simulink model "NonlinearSystemIdentificationMethod1"  (R2022b)
settings: Solver=VariableStepAuto  StartTime=0.0  StopTime=4  RelTol=0.00001
undefined symbols (not defined in the file): K, L, T, T1, T2
settings Model: Creator=amirz  LastModifiedBy=amirz

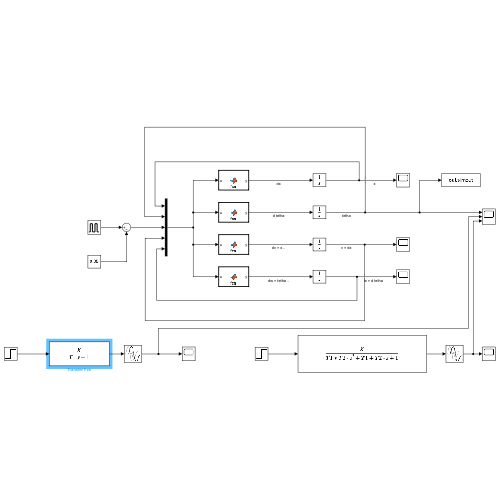
[thumbnail: Simulink's stored preview of the top-level diagram]
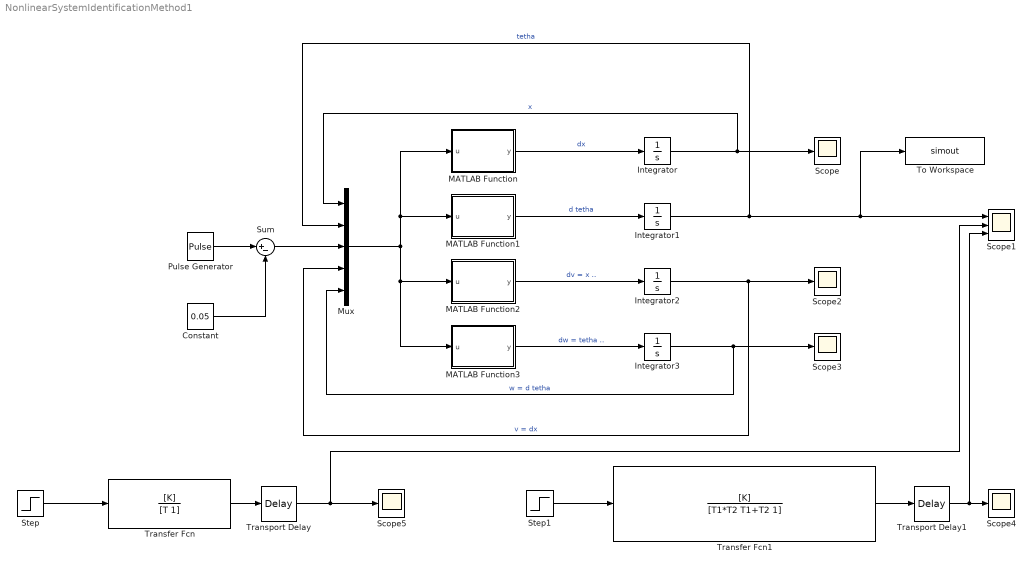
== system NonlinearSystemIdentificationMethod1 ==
  Constant : Constant  Value=0.05
  Integrator{,1..3} (4 alike) : Integrator
  MATLAB Function : MATLAB Function  TreatAsAtomicUnit=on
  MATLAB Function1 : MATLAB Function  TreatAsAtomicUnit=on
  MATLAB Function2 : MATLAB Function  TreatAsAtomicUnit=on
  MATLAB Function3 : MATLAB Function  TreatAsAtomicUnit=on
  Mux : Mux  Inputs=5
  Pulse Generator : DiscretePulseGenerator  PulseType=Time based  Amplitude=-0.1  Period=0.01  PulseWidth=50
  Scope{,2..5} (5 alike) : Scope
  Scope1 : Scope  NumInputPorts=3
  Step : Step  Time=0  SampleTime=0
  Step1 : Step  Time=0  SampleTime=0
  Sum : Sum  Inputs=|+-
  To Workspace : ToWorkspace  VariableName=simout  SaveFormat=Timeseries  SampleTime=-1
  Transfer Fcn : TransferFcn  Numerator=[K]  Denominator=[T 1]
  Transfer Fcn1 : TransferFcn  Numerator=[K]  Denominator=[T1*T2 T1+T2 1]
  Transport Delay : TransportDelay  DelayTime=L  InitialOutput=0.01
  Transport Delay1 : TransportDelay  DelayTime=L
  wires:
  MATLAB Function3/1(y) -> Integrator3/1  "dw = tetha .."
  MATLAB Function2/1(y) -> Integrator2/1  "dv = x .."
  MATLAB Function1/1(y) -> Integrator1/1  "d tetha"
  MATLAB Function/1(y) -> Integrator/1  "dx"
  Integrator3/1 -> Mux/5, Scope3/1  "w = d tetha"
  Integrator2/1 -> Mux/4, Scope2/1  "v = dx"
  Integrator1/1 -> To Workspace/1, Scope1/1, Mux/2  "tetha"
  Integrator/1 -> Mux/1, Scope/1  "x"
  Mux/1 -> MATLAB Function2/1(u), MATLAB Function3/1(u), MATLAB Function/1(u), MATLAB Function1/1(u)
  Transfer Fcn/1 -> Transport Delay/1
  Transfer Fcn1/1 -> Transport Delay1/1
  Step1/1 -> Transfer Fcn1/1
  Transport Delay/1 -> Scope1/2, Scope5/1
  Step/1 -> Transfer Fcn/1
  Sum/1 -> Mux/3
  Pulse Generator/1 -> Sum/1
  Constant/1 -> Sum/2
  Transport Delay1/1 -> Scope1/3, Scope4/1

== matlab function NonlinearSystemIdentificationMethod1/MATLAB Function ==
  data: u input size=[1,5]; y output
function y = fcn(u)
M = 10;
m = 0.3;
l = 0.3;
g = 9.8;
y = u(4);

== matlab function NonlinearSystemIdentificationMethod1/MATLAB Function2 ==
  data: u input size=[1,5]; y output
function y = fcn(u)
M = 10;
m = 0.3;
l = 0.3;
g = 9.8;
y = (u(3) + m*l*u(5)*u(5)*sin(u(2)) - m*g*sin(u(2))*cos(u(2)))/(M + m - m*cos(u(2))*cos(u(2)));

== matlab function NonlinearSystemIdentificationMethod1/MATLAB Function3 ==
  data: u input size=[1,5]; y output
function y = fcn(u)
M = 10;
m = 0.3;
l = 0.3;
g = 9.8;
y = (-u(3)*cos(u(2)) - m*l*u(5)*u(5)*sin(u(2))*cos(u(2)) + M*g*sin(u(2)) + m*g*sin(u(2)))/(l*M + l*m - l*m*cos(u(2))*cos(u(2)));

== matlab function NonlinearSystemIdentificationMethod1/MATLAB Function1 ==
  data: u input size=[1,5]; y output
function y = fcn(u)
M = 10;
m = 0.3;
l = 0.3;
g = 9.8;
y = u(5);
